simulink model "sensores_temp_testing"  (R2021a)
settings: Solver=VariableStepAuto  StartTime=0.0  StopTime=30  RelTol=1e-3
libraries: simulink x2
settings Model: Creator=Francisco  LastModifiedBy=juaco
settings SolverCC: AlgebraicLoopSolver=TrustRegion
settings OptimizationCC: LifeSpan=inf
settings DebuggingCC: SFExecutionAtInitializationDiag=none  SFMachineParentedDataDiag=warning  ArithmeticOperatorsInVariantConditions=warning
settings SFSimCC: CustomCodeUndefinedFunction=UseInterfaceOnly
settings CodeAppCC: StateflowObjectComments=on

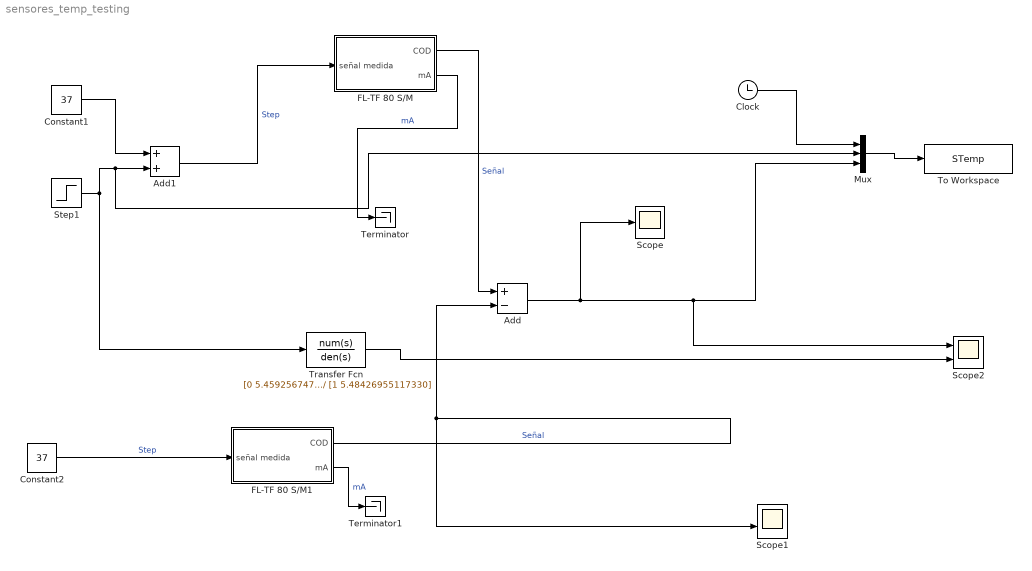
== system sensores_temp_testing ==
  Add : Sum  Inputs=+-
  Add1 : Sum
  Clock : Clock
  Constant1 : Constant  Value=37
  Constant2 : Constant  Value=37
  FL-TF 80 S/M : Subsystem  mask{To=0.001, d=0, DS=0.15, Ks=0.175, Tau=0.0000667, yo=0, Vi=37}
      mask prompts: To "Tiempo de muestreo (s)"; d "Retardo (s)"; DS "Desviacion estandar (C°)"; Ks "Sensibilidad (mA/C°)"; Tau "Constante de tiempo (s)"; yo "Sesgo (C°)"; Vi "Valor inicial (C°)"
      mask init:
      | NP=To*DS*DS;
      mask Display: image(imread('sensor5.png'))
  FL-TF 80 S/M1 : Subsystem  mask{To=0.001, d=0, DS=0.15, Ks=0.175, Tau=0.0000667, yo=0, Vi=37}
      mask prompts: To "Tiempo de muestreo (s)"; d "Retardo (s)"; DS "Desviacion estandar (C°)"; Ks "Sensibilidad (mA/C°)"; Tau "Constante de tiempo (s)"; yo "Sesgo (C°)"; Vi "Valor inicial (C°)"
      mask init:
      | NP=To*DS*DS;
      mask Display: image(imread('sensor5.png'))
  Mux : Mux  Inputs=3
  Scope : Scope
  Scope1 : Scope  NumInputPorts=4
  Scope2 : Scope  NumInputPorts=2
  Step1 : Step  Time=5  SampleTime=0
  Terminator : Terminator
  Terminator1 : Terminator
  To Workspace : ToWorkspace  VariableName=STemp  SampleTime=-1
  Transfer Fcn : TransferFcn  Numerator=[0 5.45925674729626]  Denominator=[1 5.48426955117330]
  wires:
  Step1/1 -> Mux/2, Add1/2, Transfer Fcn/1
  Add1/1 -> FL-TF 80 S/M/1(señal medida)  "Step"
  Constant1/1 -> Add1/1
  FL-TF 80 S/M/2(mA) -> Terminator/1  "mA"
  FL-TF 80 S/M/1(COD) -> Add/1  "Señal"
  Clock/1 -> Mux/1
  Mux/1 -> To Workspace/1
  FL-TF 80 S/M1/1(COD) -> Add/2, Scope1/3  "Señal"
  Constant2/1 -> FL-TF 80 S/M1/1(señal medida)  "Step"
  FL-TF 80 S/M1/2(mA) -> Terminator1/1  "mA"
  Add/1 -> Scope/1, Scope2/1, Mux/3
  Transfer Fcn/1 -> Scope2/2

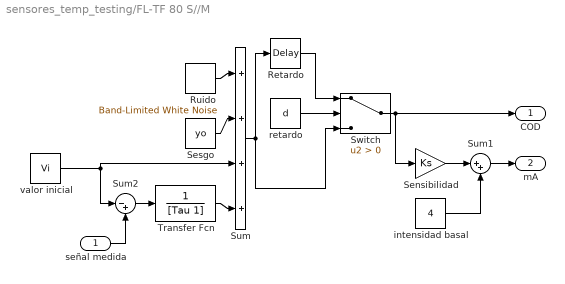
== system sensores_temp_testing/FL-TF 80 S//M ==
  señal medida : Inport
  Retardo : TransportDelay  DelayTime=d
  Ruido : simulink/Sources/Band-Limited White Noise  Cov=[NP]  Ts=To  seed=[23341]
  Sensibilidad : Gain  Gain=Ks
  Sesgo : Constant  Value=yo
  Sum : Sum  Inputs=|++++  SaturateOnIntegerOverflow=on
  Sum1 : Sum  Inputs=|++
  Sum2 : Sum  Inputs=|-+
  Switch : Switch  Criteria=u2 > Threshold
  Transfer Fcn : TransferFcn  Denominator=[Tau 1]
  intensidad basal : Constant  Value=4
  retardo : Constant  Value=d
  valor inicial : Constant  Value=Vi
  COD : Outport
  mA : Outport  Port=2
  wires:
  Sensibilidad/1 -> Sum1/1
  Sum1/1 -> mA/1
  intensidad basal/1 -> Sum1/2
  retardo/1 -> Switch/2
  Sum/1 -> Retardo/1, Switch/3
  Retardo/1 -> Switch/1
  Switch/1 -> COD/1, Sensibilidad/1
  Sesgo/1 -> Sum/2
  Ruido/1 -> Sum/1
  Transfer Fcn/1 -> Sum/4
  Sum2/1 -> Transfer Fcn/1
  señal medida/1 -> Sum2/2
  valor inicial/1 -> Sum/3, Sum2/1

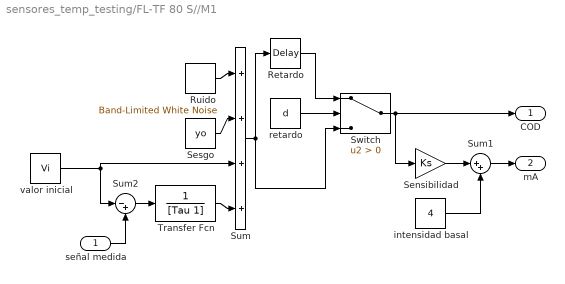
== system sensores_temp_testing/FL-TF 80 S//M1 ==
  señal medida : Inport
  Retardo : TransportDelay  DelayTime=d
  Ruido : simulink/Sources/Band-Limited White Noise  Cov=[NP]  Ts=To  seed=[23341]
  Sensibilidad : Gain  Gain=Ks
  Sesgo : Constant  Value=yo
  Sum : Sum  Inputs=|++++  SaturateOnIntegerOverflow=on
  Sum1 : Sum  Inputs=|++
  Sum2 : Sum  Inputs=|-+
  Switch : Switch  Criteria=u2 > Threshold
  Transfer Fcn : TransferFcn  Denominator=[Tau 1]
  intensidad basal : Constant  Value=4
  retardo : Constant  Value=d
  valor inicial : Constant  Value=Vi
  COD : Outport
  mA : Outport  Port=2
  wires:
  Sensibilidad/1 -> Sum1/1
  Sum1/1 -> mA/1
  intensidad basal/1 -> Sum1/2
  retardo/1 -> Switch/2
  Sum/1 -> Retardo/1, Switch/3
  Retardo/1 -> Switch/1
  Switch/1 -> COD/1, Sensibilidad/1
  Sesgo/1 -> Sum/2
  Ruido/1 -> Sum/1
  Transfer Fcn/1 -> Sum/4
  Sum2/1 -> Transfer Fcn/1
  señal medida/1 -> Sum2/2
  valor inicial/1 -> Sum/3, Sum2/1
